simulink model "Q2a"  (R2023b)
settings: Solver=FixedStepAuto  StartTime=0.0  StopTime=90  FixedStep=0.01  RelTol=1e-3
undefined symbols (not defined in the file or in its folder): Continuous, Time
libraries: ctrlSharedLib x1
settings Model: Creator=Ali  LastModifiedBy=Ali

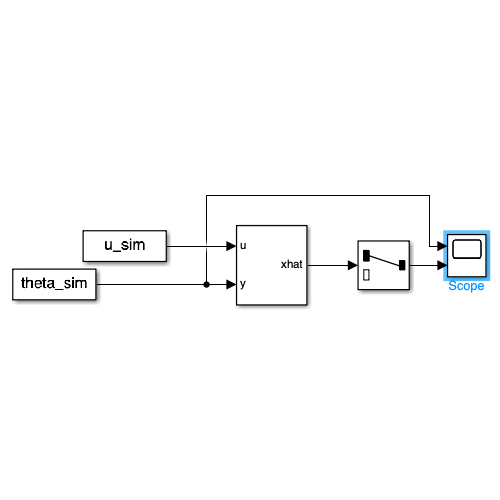
[thumbnail: Simulink's stored preview of the top-level diagram]
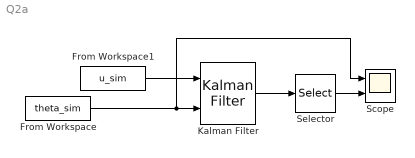
== system Q2a ==
  From Workspace : FromWorkspace  VariableName=theta_sim
  From Workspace1 : FromWorkspace  VariableName=u_sim
  Kalman Filter : ctrlSharedLib/Kalman Filter  TimeDomain=Continuous-Time  UseCurrentEstimator=on  ModelSource=Individual A, B, C, D matrices  ModelSourceVariable=ss(0.95,1,1,0,1)  A=[0 1; 0 0]  B=[0; 0.72]  C=[1, 0]  D=0  NumberOfStates=1  NumberOfInputs=1  NumberOfOutputs=1  InitialEstimateSource=Dialog  X0=0  P0=10  UseK=off  UseGH=off  NumberOfProcessNoiseInputs=1  G=1  TimeInvariantG=on  H=0  TimeInvariantH=on  Q=0.5  TimeInvariantQ=on  R=1  TimeInvariantR=on  N=0  TimeInvariantN=on  AddInputPort=on  AddEnablePort=off  OutputEstimatedY=off  OutputP=off  Ts=-1
  Scope : Scope  NumInputPorts=2
  Selector : Selector  InputPortWidth=2  IndexOptions=Index vector (dialog)  Indices=[1]  OutputSizes=1
  wires:
  From Workspace/1 -> Scope/1, Kalman Filter/2
  From Workspace1/1 -> Kalman Filter/1
  Kalman Filter/1 -> Selector/1
  Selector/1 -> Scope/2
